simulink model "PSO_ZVD"  (R2021a)
settings: Solver=VariableStepAuto  StartTime=0.0  StopTime=20  RelTol=1e-3
InitFcn:
  | ml=2;
  | 
  | mc=0.5;
  | M2=0.5;
  | 
  | mt=5;
  | g=9.81;
  | l_ref=0.1;
  | l_ini=1;
  | l=l_ini;
  | x_ref=1;
  | n1=5;n2=1;
  | 
  | %ADRC' s parameter caculation
  | %b0 = (ml+mc)/(mc*ml +mc*mt+ml*mt); %Hieu
  | b0=(ml+mc)/(mt*mc+2*ml*mc+mt*ml+ml^2+mc^2); %Enhanced-coupling
  | k_ESO = 100;
  | T_set  = 6;
  | 
  | s_cl = -5.85/T_set;
  | Kp   = s_cl^2;
  | Kd   = -2*s_cl;
  | 
  | s_ESO = k_ESO*s_cl;
  | l1        = -3*s_ESO;
  | l2        = 3*( s_ESO)^2;
  | l3        = -(s_ESO)^3;
  | 
  | %b1 = (mt+mc)/(mc*ml +mc*mt+ml*mt);
  | b1=1/(ml+mc);
  | k_ESO1 =100;
  | T_set1  = 3;
  | s_cl1 = -5.85/T_set1;
  | Kp1   = s_cl1^2;
  | Kd1   = -2*s_cl1;
  | 
  | s_ESO1 = k_ESO1*s_cl1;
  | l11        = -3*s_ESO1;
  | l21        = 3*( s_ESO1)^2;
  | l31        = -(s_ESO1)^3;
  | 
  | 
  | L1=l_ini;
  | %L2=0.5;
  | L2=0.1;
  | m1=2;
  | m2=mc;
  | m=5;
  | %Bo input shaping
  | alpha = (1/L1 + 1/L2)*(m1+M2)/m1;
  | beta = (((m1+M2)/m1)^2)*((1/L1 + 1/L2)^2) - 4*(m1+M2)/(m1*L1*L2);
  | w1 = sqrt(g*(alpha - sqrt(beta))/2);
  | w2 = sqrt(g*(alpha + sqrt(beta))/2);
  | damping_ratio = 0;
  | wd1 = w1*sqrt(1-damping_ratio^2);
  | wd2 = w2*sqrt(1-damping_ratio^2);
  | k = exp(damping_ratio*pi/sqrt(1-damping_ratio^2));
  | 
  | %ZVD1
  | t1_ZVD_1=pi/wd1;
  | ... (+27 lines)
values from neighbouring files (symbols this model uses):
  particle = repmat(empty_particle, nPop, 1)    [PSO16_12.m]    (also in PSO_ZVD.m)
undefined symbols (not defined in the file or in its folder): i, li, xi
libraries: neural x101, simulink_extras x13, simulink x3
(part 23 of 34)

== matlab function PSO_ZVD/non linear model/con lắc đôi4/Crane ==
  data: dx1 output; d1x input; l1 input; d1l1 input; the1 input; d1the1 input; the2 input; d1the2 input; Fx input; Fl input; dx2 output; dx3 output; dx4 output; dx5 output; dx6 output; m2 input; dx7 output; dx8 output
function [dx1,dx2,dx3,dx4,dx5,dx6,dx7,dx8] = fcn(d1x,l1,d1l1,the1,d1the1,the2,d1the2,Fx,Fl,m2)
 m =5; m1 =2; g =9.81; l2=0.5;bx=82; bl=50;bc=0.1;

 dx1=d1x;

 dx2 =(Fx*l1*l2*m2*cos(the1 - the2)^2 - Fx*l1*l2*m2 - d1the2^2*l1*l2^2*m2^2*sin(the2) - Fx*l1*l2*m1 + Fx*l1*l2*m2*sin(the1 - the2)^2 + bx*d1x*l1*l2*m1 + bx*d1x*l1*l2*m2 + Fl*l1*l2*m1*sin(the1) + Fl*l1*l2*m2*sin(the1) - bc*d1the1*l2*m1*cos(the1) - bc*d1the1*l2*m2*cos(the1) - bc*d1the2*l1*m1*cos(the2) - bc*d1the2*l1*m2*cos(the2) + bc*d1the2*l1*m1*sin(the1 - the2)*sin(the1) + bc*d1the2*l1*m2*sin(the1 - the2)*sin(the1) + d1the2^2*l1*l2^2*m2^2*cos(the1 - the2)*sin(the1) - d1the2^2*l1*l2^2*m2^2*sin(the1 - the2)*cos(the1) - d1the2^2*l1*l2^2*m1*m2*sin(the2) - g*l1*l2*m2^2*cos(the2)*sin(the2) - Fl*l1*l2*m2*cos(the1 - the2)^2*sin(the1) + bc*d1the1*l2*m2*sin(the1 - the2)^2*cos(the1) - bl*d1l1*l1*l2*m1*sin(the1) - bl*d1l1*l1*l2*m2*sin(the1) + d1the2^2*l1*l2^2*m2^2*cos(the1 - the2)^2*sin(the2) - d1the2^2*l1*l2^2*m2^2*cos(the1 - the2)^3*sin(the1) + d1the2^2*l1*l2^2*m2^2*sin(the1 - the2)^3*cos(the1) + d1the2^2*l1*l2^2*m2^2*sin(the1 - the2)^2*sin(the2) - bx*d1x*l1*l2*m2*cos(the1 - the2)^2 - Fl*l1*l2*m2*sin(the1 - the2)*cos(the2) + bc*d1the2*l1*m1*cos(the1 - the2)*cos(the1) + bc*d1the2*l1*m2*cos(the1 - the2)*cos(the1) + bc*d1the1*l2*m2*cos(the1 - the2)*cos(the2) - bx*d1x*l1*l2*m2*sin(the1 - the2)^2 - bc*d1the1*l2*m2*cos(the1 - the2)*sin(the1 - the2)*sin(the1) + d1the2^2*l1*l2^2*m1*m2*cos(the1 - the2)*sin(the1) - d1the2^2*l1*l2^2*m1*m2*sin(the1 - the2)*cos(the1) + g*l1*l2*m2^2*cos(the1 - the2)*cos(the1)*sin(the2) + g*l1*l2*m2^2*cos(the1 - the2)*cos(the2)*sin(the1) - g*l1*l2*m2^2*sin(the1 - the2)*cos(the1)*cos(the2) - g*l1*l2*m1*m2*cos(the2)*sin(the2) + g*l1*l2*m2^2*sin(the1 - the2)*sin(the1)*sin(the2) + bl*d1l1*l1*l2*m2*sin(the1 - the2)*cos(the2) + d1the2^2*l1*l2^2*m2^2*cos(the1 - the2)^2*sin(the1 - the2)*cos(the1) - d1the2^2*l1*l2^2*m2^2*cos(the1 - the2)*sin(the1 - the2)^2*sin(the1) - g*l1*l2*m2^2*cos(the1 - the2)^2*cos(the1)*sin(the1) + g*l1*l2*m2^2*sin(the1 - the2)^2*cos(the1)*sin(the1) + bl*d1l1*l1*l2*m2*cos(the1 - the2)^2*sin(the1) + g*l1*l2*m2^2*cos(the1 - the2)*sin(the1 - the2)*cos(the1)^2 - g*l1*l2*m2^2*cos(the1 - the2)*sin(the1 - the2)*sin(the1)^2 + Fl*l1*l2*m2*cos(the1 - the2)*sin(the1 - the2)*cos(the1) + g*l1*l2*m1*m2*cos(the1 - the2)*cos(the1)*sin(the2) + g*l1*l2*m1*m2*cos(the1 - the2)*cos(the2)*sin(the1) - g*l1*l2*m1*m2*sin(the1 - the2)*cos(the1)*cos(the2) + g*l1*l2*m1*m2*sin(the1 - the2)*sin(the1)*sin(the2) - bl*d1l1*l1*l2*m2*cos(the1 - the2)*sin(the1 - the2)*cos(the1) - g*l1*l2*m1*m2*cos(the1 - the2)^2*cos(the1)*sin(the1) + g*l1*l2*m1*m2*sin(the1 - the2)^2*cos(the1)*sin(the1) + g*l1*l2*m1*m2*cos(the1 - the2)*sin(the1 - the2)*cos(the1)^2 - g*l1*l2*m1*m2*cos(the1 - the2)*sin(the1 - the2)*sin(the1)^2)/(l1*l2*(m1^2*cos(the1)^2 - m*m2 - 2*m1*m2 - m*m1 + m2^2*cos(the1)^2 + m2^2*cos(the2)^2 + m1^2*sin(the1)^2 + m2^2*sin(the1)^2 + m2^2*cos(the1 - the2)^2 + m2^2*sin(the1 - the2)^2 - m1^2 - m2^2 + 2*m1*m2*cos(the1)^2 + m1*m2*cos(the2)^2 + 2*m1*m2*sin(the1)^2 + m*m2*cos(the1 - the2)^2 + m1*m2*cos(the1 - the2)^2 + m*m2*sin(the1 - the2)^2 + m1*m2*sin(the1 - the2)^2 - m2^2*cos(the1 - the2)^2*sin(the1)^2 - m2^2*sin(the1 - the2)^2*cos(the1)^2 - 2*m2^2*sin(the1 - the2)*cos(the2)*sin(the1) - 2*m2^2*cos(the1 - the2)*cos(the1)*cos(the2) - m1*m2*cos(the1 - the2)^2*sin(the1)^2 - m1*m2*sin(the1 - the2)^2*cos(the1)^2 + 2*m2^2*cos(the1 - the2)*sin(the1 - the2)*cos(the1)*sin(the1) - 2*m1*m2*sin(the1 - the2)*cos(the2)*sin(the1) - 2*m1*m2*cos(the1 - the2)*cos(the1)*cos(the2) + 2*m1*m2*cos(the1 - the2)*sin(the1 - the2)*cos(the1)*sin(the1)));

 dx3=d1l1;

 dx4 = (Fx*l1*l2*m1^2*sin(the1) - d1the1^2*l1^2*l2*m2^3 - Fl*l1*l2*m1^2 - Fl*l1*l2*m2^2 - d1the2^2*l1*l2^2*m2^3*cos(the1 - the2) - d1the1^2*l1^2*l2*m1^3 + Fx*l1*l2*m2^2*sin(the1) - g*l1*l2*m1^3*cos(the1) - g*l1*l2*m2^3*cos(the1) - Fl*l1*l2*m*m1 - Fl*l1*l2*m*m2 - 2*Fl*l1*l2*m1*m2 + d1the1^2*l1^2*l2*m1^3*cos(the1)^2 + d1the1^2*l1^2*l2*m2^3*cos(the1)^2 + d1the1^2*l1^2*l2*m2^3*cos(the2)^2 + d1the1^2*l1^2*l2*m1^3*sin(the1)^2 + d1the1^2*l1^2*l2*m2^3*sin(the1)^2 - bc*d1the2*l1*m1^2*sin(the1 - the2) - bc*d1the2*l1*m2^2*sin(the1 - the2) + Fl*l1*l2*m1^2*cos(the1)^2 + Fl*l1*l2*m2^2*cos(the1)^2 + Fl*l1*l2*m2^2*cos(the2)^2 + d1the1^2*l1^2*l2*m2^3*cos(the1 - the2)^2 + d1the2^2*l1*l2^2*m2^3*cos(the1 - the2)^3 - d1the1^2*l1^2*l2*m*m1^2 - d1the1^2*l1^2*l2*m*m2^2 - 3*d1the1^2*l1^2*l2*m1*m2^2 - 3*d1the1^2*l1^2*l2*m1^2*m2 + d1the1^2*l1^2*l2*m2^3*sin(the1 - the2)^2 + g*l1*l2*m1^3*cos(the1)^3 + g*l1*l2*m2^3*cos(the1)^3 + Fl*l1*l2*m2^2*cos(the1 - the2)^2 + bl*d1l1*l1*l2*m1^2 + bl*d1l1*l1*l2*m2^2 - bl*d1l1*l1*l2*m1^2*cos(the1)^2 - bl*d1l1*l1*l2*m2^2*cos(the1)^2 - bl*d1l1*l1*l2*m2^2*cos(the2)^2 + d1the1^2*l1^2*l2*m*m2^2*sin(the1 - the2)^2 + 2*d1the1^2*l1^2*l2*m1*m2^2*sin(the1 - the2)^2 + d1the1^2*l1^2*l2*m1^2*m2*sin(the1 - the2)^2 + 3*g*l1*l2*m1*m2^2*cos(the1)^3 + 3*g*l1*l2*m1^2*m2*cos(the1)^3 + bc*d1the1*l2*m1^2*cos(the1)*sin(the1) + bc*d1the1*l2*m2^2*cos(the1)*sin(the1) + bc*d1the2*l1*m1^2*cos(the2)*sin(the1) + bc*d1the2*l1*m2^2*cos(the2)*sin(the1) - bl*d1l1*l1*l2*m2^2*cos(the1 - the2)^2 - Fx*l1*l2*m2^2*sin(the1 - the2)*cos(the2) + 2*Fx*l1*l2*m1*m2*sin(the1) + d1the2^2*l1*l2^2*m2^3*cos(the1 - the2)*cos(the1)^2 + d1the2^2*l1*l2^2*m2^3*cos(the1 - the2)*cos(the2)^2 - g*l1*l2*m2^3*sin(the1 - the2)*sin(the2) + g*l1*l2*m2^3*cos(the1)*cos(the2)^2 + bc*d1the1*l2*m2^2*cos(the1 - the2)*sin(the1 - the2) - bc*d1the2*l1*m*m1*sin(the1 - the2) - bc*d1the2*l1*m*m2*sin(the1 - the2) - 2*bc*d1the2*l1*m1*m2*sin(the1 - the2) + g*l1*l2*m1^3*cos(the1)*sin(the1)^2 + g*l1*l2*m2^3*cos(the1)*sin(the1)^2 + 2*Fl*l1*l2*m1*m2*cos(the1)^2 + Fl*l1*l2*m1*m2*cos(the2)^2 - Fx*l1*l2*m2^2*cos(the1 - the2)^2*sin(the1) - d1the2^2*l1*l2^2*m*m2^2*cos(the1 - the2) - 2*d1the2^2*l1*l2^2*m1*m2^2*cos(the1 - the2) - d1the2^2*l1*l2^2*m1^2*m2*cos(the1 - the2) - 2*d1the1^2*l1^2*l2*m*m1*m2 + d1the2^2*l1*l2^2*m2^3*cos(the1 - the2)*sin(the1 - the2)^2 + g*l1*l2*m2^3*cos(the1 - the2)^2*cos(the1) - g*l1*l2*m*m1^2*cos(the1) - g*l1*l2*m*m2^2*cos(the1) - 3*g*l1*l2*m1*m2^2*cos(the1) - 3*g*l1*l2*m1^2*m2*cos(the1) + bc*d1the2*l1*m1^2*sin(the1 - the2)*cos(the1)^2 + bc*d1the2*l1*m2^2*sin(the1 - the2)*cos(the1)^2 - bx*d1x*l1*l2*m1^2*sin(the1) - bx*d1x*l1*l2*m2^2*sin(the1) + Fl*l1*l2*m*m2*cos(the1 - the2)^2 + Fl*l1*l2*m1*m2*cos(the1 - the2)^2 + 3*d1the1^2*l1^2*l2*m1*m2^2*cos(the1)^2 + 3*d1the1^2*l1^2*l2*m1^2*m2*cos(the1)^2 + 2*d1the1^2*l1^2*l2*m1*m2^2*cos(the2)^2 + d1the1^2*l1^2*l2*m1^2*m2*cos(the2)^2 + bl*d1l1*l1*l2*m*m1 + bl*d1l1*l1*l2*m*m2 + 2*bl*d1l1*l1*l2*m1*m2 - d1the1^2*l1^2*l2*m2^3*cos(the1 - the2)^2*sin(the1)^2 - d1the1^2*l1^2*l2*m2^3*sin(the1 - the2)^2*cos(the1)^2 + 3*d1the1^2*l1^2*l2*m1*m2^2*sin(the1)^2 + 3*d1the1^2*l1^2*l2*m1^2*m2*sin(the1)^2 + d1the2^2*l1*l2^2*m2^3*sin(the1)*sin(the2) + d1the1^2*l1^2*l2*m*m2^2*cos(the1 - the2)^2 + 2*d1the1^2*l1^2*l2*m1*m2^2*cos(the1 - the2)^2 + d1the1^2*l1^2*l2*m1^2*m2*cos(the1 - the2)^2 + d1the2^2*l1*l2^2*m*m2^2*cos(the1 - the2)^3 + d1the2^2*l1*l2^2*m1*m2^2*cos(the1 - the2)^3 - 2*d1the1^2*l1^2*l2*m2^3*sin(the1 - the2)*cos(the2)*sin(the1) + d1the2^2*l1*l2^2*m2^3*sin(the1 - the2)*cos(the1)*sin(the1) - d1the2^2*l1*l2^2*m2^3*sin(the1 - the2)*cos(the2)*sin(the2) - 2*Fl*l1*l2*m2^2*cos(the1 - the2)*cos(the1)*cos(the2) + d1the1^2*l1^2*l2*m*m1*m2*cos(the1 - the2)^2 - 2*bl*d1l1*l1*l2*m1*m2*cos(the1)^2 - bl*d1l1*l1*l2*m1*m2*cos(the2)^2 + g*l1*l2*m2^3*cos(the2)*sin(the1)*sin(the2) + d1the2^2*l1*l2^2*m*m2^2*cos(the1 - the2)*sin(the1 - the2)^2 + d1the2^2*l1*l2^2*m1*m2^2*cos(the1 - the2)*sin(the1 - the2)^2 + g*l1*l2*m*m2^2*cos(the1 - the2)^2*cos(the1) + 2*g*l1*l2*m1*m2^2*cos(the1 - the2)^2*cos(the1) + g*l1*l2*m1^2*m2*cos(the1 - the2)^2*cos(the1) + d1the1^2*l1^2*l2*m*m1*m2*sin(the1 - the2)^2 + bx*d1x*l1*l2*m2^2*cos(the1 - the2)^2*sin(the1) - bc*d1the2*l1*m1^2*cos(the1 - the2)*cos(the1)*sin(the1) - bc*d1the2*l1*m2^2*cos(the1 - the2)*cos(the1)*sin(the1) - bc*d1the1*l2*m2^2*cos(the1 - the2)*cos(the2)*sin(the1) - bc*d1the1*l2*m2^2*sin(the1 - the2)*cos(the1)*cos(the2) + 2*bc*d1the1*l2*m1*m2*cos(the1)*sin(the1) + 2*bc*d1the2*l1*m1*m2*cos(the2)*sin(the1) - 2*d1the2^2*l1*l2^2*m2^3*cos(the1 - the2)^2*cos(the1)*cos(the2) - bl*d1l1*l1*l2*m*m2*cos(the1 - the2)^2 - bl*d1l1*l1*l2*m1*m2*cos(the1 - the2)^2 - 2*d1the1^2*l1^2*l2*m1*m2^2*cos(the1 - the2)^2*sin(the1)^2 - 2*d1the1^2*l1^2*l2*m1*m2^2*sin(the1 - the2)^2*cos(the1)^2 - d1the1^2*l1^2*l2*m1^2*m2*cos(the1 - the2)^2*sin(the1)^2 - d1the1^2*l1^2*l2*m1^2*m2*sin(the1 - the2)^2*cos(the1)^2 + Fx*l1*l2*m2^2*cos(the1 - the2)*sin(the1 - the2)*cos(the1) - Fx*l1*l2*m1*m2*sin(the1 - the2)*cos(the2) - d1the2^2*l1*l2^2*m2^3*sin(the1 - the2)^2*cos(the1)*cos(the2) - d1the2^2*l1*l2^2*m2^3*cos(the1 - the2)^2*sin(the1)*sin(the2) + 2*d1the2^2*l1*l2^2*m1*m2^2*sin(the1)*sin(the2) + d1the2^2*l1*l2^2*m1^2*m2*sin(the1)*sin(the2) + g*l1*l2*m2^3*cos(the1 - the2)*sin(the1 - the2)*sin(the1) - 2*g*l1*l2*m2^3*cos(the1 - the2)*cos(the1)^2*cos(the2) + bc*d1the1*l2*m*m2*cos(the1 - the2)*sin(the1 - the2) + bc*d1the1*l2*m1*m2*cos(the1 - the2)*sin(the1 - the2) - g*l1*l2*m2^3*cos(the1 - the2)*cos(the2)*sin(the1)^2 + g*l1*l2*m2^3*sin(the1 - the2)*cos(the1)^2*sin(the2) - Fx*l1*l2*m1*m2*cos(the1 - the2)^2*sin(the1) - d1the2^2*l1*l2^2*m*m1*m2*cos(the1 - the2) - 2*g*l1*l2*m*m1*m2*cos(the1) + bx*d1x*l1*l2*m2^2*sin(the1 - the2)*cos(the2) + 2*bc*d1the2*l1*m1*m2*sin(the1 - the2)*cos(the1)^2 - 2*bx*d1x*l1*l2*m1*m2*sin(the1) + 2*d1the2^2*l1*l2^2*m1*m2^2*cos(the1 - the2)*cos(the1)^2 + d1the2^2*l1*l2^2*m1^2*m2*cos(the1 - the2)*cos(the1)^2 + d1the2^2*l1*l2^2*m1*m2^2*cos(the1 - the2)*cos(the2)^2 - g*l1*l2*m*m2^2*sin(the1 - the2)*sin(the2) - 2*g*l1*l2*m1*m2^2*sin(the1 - the2)*sin(the2) - g*l1*l2*m1^2*m2*sin(the1 - the2)*sin(the2) - 2*d1the1^2*l1^2*l2*m2^3*cos(the1 - the2)*cos(the1)*cos(the2) + 2*g*l1*l2*m1*m2^2*cos(the1)*cos(the2)^2 + g*l1*l2*m1^2*m2*cos(the1)*cos(the2)^2 + 3*g*l1*l2*m1*m2^2*cos(the1)*sin(the1)^2 + 3*g*l1*l2*m1^2*m2*cos(the1)*sin(the1)^2 - 2*g*l1*l2*m1*m2^2*cos(the1 - the2)*cos(the2)*sin(the1)^2 - g*l1*l2*m1^2*m2*cos(the1 - the2)*cos(the2)*sin(the1)^2 + 2*d1the1^2*l1^2*l2*m2^3*cos(the1 - the2)*sin(the1 - the2)*cos(the1)*sin(the1) + d1the2^2*l1*l2^2*m2^3*cos(the1 - the2)*sin(the1 - the2)*cos(the1)*sin(the2) - d1the2^2*l1*l2^2*m2^3*cos(the1 - the2)*sin(the1 - the2)*cos(the2)*sin(the1) + 2*g*l1*l2*m1*m2^2*sin(the1 - the2)*cos(the1)^2*sin(the2) + g*l1*l2*m1^2*m2*sin(the1 - the2)*cos(the1)^2*sin(the2) - 2*Fl*l1*l2*m1*m2*cos(the1 - the2)*cos(the1)*cos(the2) - g*l1*l2*m2^3*cos(the1 - the2)*cos(the1)*sin(the1)*sin(the2) - g*l1*l2*m2^3*sin(the1 - the2)*cos(the1)*cos(the2)*sin(the1) + g*l1*l2*m*m1*m2*cos(the1 - the2)^2*cos(the1) + bx*d1x*l1*l2*m1*m2*cos(the1 - the2)^2*sin(the1) - 2*bc*d1the2*l1*m1*m2*cos(the1 - the2)*cos(the1)*sin(the1) - bc*d1the1*l2*m1*m2*cos(the1 - the2)*cos(the2)*sin(the1) - bc*d1the1*l2*m1*m2*sin(the1 - the2)*cos(the1)*cos(the2) - 4*d1the1^2*l1^2*l2*m1*m2^2*cos(the1 - the2)*cos(the1)*cos(the2) - 2*d1the1^2*l1^2*l2*m1^2*m2*cos(the1 - the2)*cos(the1)*cos(the2) + Fx*l1*l2*m1*m2*cos(the1 - the2)*sin(the1 - the2)*cos(the1) - 4*d1the1^2*l1^2*l2*m1*m2^2*sin(the1 - the2)*cos(the2)*sin(the1) - 2*d1the1^2*l1^2*l2*m1^2*m2*sin(the1 - the2)*cos(the2)*sin(the1) + 2*d1the2^2*l1*l2^2*m1*m2^2*sin(the1 - the2)*cos(the1)*sin(the1) + d1the2^2*l1*l2^2*m1^2*m2*sin(the1 - the2)*cos(the1)*sin(the1) - d1the2^2*l1*l2^2*m1*m2^2*sin(the1 - the2)*cos(the2)*sin(the2) + 2*g*l1*l2*m1*m2^2*cos(the2)*sin(the1)*sin(the2) + g*l1*l2*m1^2*m2*cos(the2)*sin(the1)*sin(the2) + 2*bl*d1l1*l1*l2*m2^2*cos(the1 - the2)*cos(the1)*cos(the2) - 2*d1the2^2*l1*l2^2*m1*m2^2*cos(the1 - the2)^2*cos(the1)*cos(the2) - d1the2^2*l1*l2^2*m1*m2^2*sin(the1 - the2)^2*cos(the1)*cos(the2) - bx*d1x*l1*l2*m2^2*cos(the1 - the2)*sin(the1 - the2)*cos(the1) + bx*d1x*l1*l2*m1*m2*sin(the1 - the2)*cos(the2) - d1the2^2*l1*l2^2*m1*m2^2*cos(the1 - the2)^2*sin(the1)*sin(the2) + g*l1*l2*m*m2^2*cos(the1 - the2)*sin(the1 - the2)*sin(the1) + 2*g*l1*l2*m1*m2^2*cos(the1 - the2)*sin(the1 - the2)*sin(the1) + g*l1*l2*m1^2*m2*cos(the1 - the2)*sin(the1 - the2)*sin(the1) - g*l1*l2*m*m1*m2*sin(the1 - the2)*sin(the2) - 4*g*l1*l2*m1*m2^2*cos(the1 - the2)*cos(the1)^2*cos(the2) - 2*g*l1*l2*m1^2*m2*cos(the1 - the2)*cos(the1)^2*cos(the2) + 4*d1the1^2*l1^2*l2*m1*m2^2*cos(the1 - the2)*sin(the1 - the2)*cos(the1)*sin(the1) + 2*d1the1^2*l1^2*l2*m1^2*m2*cos(the1 - the2)*sin(the1 - the2)*cos(the1)*sin(the1) + d1the2^2*l1*l2^2*m1*m2^2*cos(the1 - the2)*sin(the1 - the2)*cos(the1)*sin(the2) - d1the2^2*l1*l2^2*m1*m2^2*cos(the1 - the2)*sin(the1 - the2)*cos(the2)*sin(the1) - 2*g*l1*l2*m1*m2^2*cos(the1 - the2)*cos(the1)*sin(the1)*sin(the2) - 2*g*l1*l2*m1*m2^2*sin(the1 - the2)*cos(the1)*cos(the2)*sin(the1) - g*l1*l2*m1^2*m2*cos(the1 - the2)*cos(the1)*sin(the1)*sin(the2) - g*l1*l2*m1^2*m2*sin(the1 - the2)*cos(the1)*cos(the2)*sin(the1) + 2*bl*d1l1*l1*l2*m1*m2*cos(the1 - the2)*cos(the1)*cos(the2) - bx*d1x*l1*l2*m1*m2*cos(the1 - the2)*sin(the1 - the2)*cos(the1) + g*l1*l2*m*m1*m2*cos(the1 - the2)*sin(the1 - the2)*sin(the1))/(l1*l2*(m1 + m2)*(m1^2*cos(the1)^2 - m*m2 - 2*m1*m2 - m*m1 + m2^2*cos(the1)^2 + m2^2*cos(the2)^2 + m1^2*sin(the1)^2 + m2^2*sin(the1)^2 + m2^2*cos(the1 - the2)^2 + m2^2*sin(the1 - the2)^2 - m1^2 - m2^2 + 2*m1*m2*cos(the1)^2 + m1*m2*cos(the2)^2 + 2*m1*m2*sin(the1)^2 + m*m2*cos(the1 - the2)^2 + m1*m2*cos(the1 - the2)^2 + m*m2*sin(the1 - the2)^2 + m1*m2*sin(the1 - the2)^2 - m2^2*cos(the1 - the2)^2*sin(the1)^2 - m2^2*sin(the1 - the2)^2*cos(the1)^2 - 2*m2^2*sin(the1 - the2)*cos(the2)*sin(the1) - 2*m2^2*cos(the1 - the2)*cos(the1)*cos(the2) - m1*m2*cos(the1 - the2)^2*sin(the1)^2 - m1*m2*sin(the1 - the2)^2*cos(the1)^2 + 2*m2^2*cos(the1 - the2)*sin(the1 - the2)*cos(the1)*sin(the1) - 2*m1*m2*sin(the1 - the2)*cos(the2)*sin(the1) - 2*m1*m2*cos(the1 - the2)*cos(the1)*cos(the2) + 2*m1*m2*cos(the1 - the2)*sin(the1 - the2)*cos(the1)*sin(the1)));

 dx5=d1the1;

 dx6 = -(bc*d1the2*l1*m1^2*cos(the1 - the2) - bc*d1the1*l2*m2^2 - Fx*l1*l2*m1^2*cos(the1) - Fx*l1*l2*m2^2*cos(the1) - d1the2^2*l1*l2^2*m2^3*sin(the1 - the2) - g*l1*l2*m1^3*sin(the1) - g*l1*l2*m2^3*sin(the1) - bc*d1the1*l2*m1^2 + bc*d1the2*l1*m2^2*cos(the1 - the2) - bc*d1the1*l2*m*m1 - bc*d1the1*l2*m*m2 - 2*bc*d1the1*l2*m1*m2 + bc*d1the1*l2*m2^2*cos(the2)^2 + d1the2^2*l1*l2^2*m2^3*sin(the1 - the2)^3 + bc*d1the1*l2*m1^2*sin(the1)^2 + bc*d1the1*l2*m2^2*sin(the1)^2 + g*l1*l2*m1^3*sin(the1)^3 + g*l1*l2*m2^3*sin(the1)^3 - 2*d1l1*d1the1*l1*l2*m1^3 - 2*d1l1*d1the1*l1*l2*m2^3 + bc*d1the1*l2*m2^2*sin(the1 - the2)^2 + 2*d1l1*d1the1*l1*l2*m1^3*cos(the1)^2 + 2*d1l1*d1the1*l1*l2*m2^3*cos(the1)^2 + 2*d1l1*d1the1*l1*l2*m2^3*cos(the2)^2 + Fl*l1*l2*m1^2*cos(the1)*sin(the1) + Fl*l1*l2*m2^2*cos(the1)*sin(the1) - bc*d1the2*l1*m1^2*cos(the1)*cos(the2) - bc*d1the2*l1*m2^2*cos(the1)*cos(the2) + d1the2^2*l1*l2^2*m*m2^2*sin(the1 - the2)^3 + d1the2^2*l1*l2^2*m1*m2^2*sin(the1 - the2)^3 + 2*d1l1*d1the1*l1*l2*m1^3*sin(the1)^2 + 2*d1l1*d1the1*l1*l2*m2^3*sin(the1)^2 + 3*g*l1*l2*m1*m2^2*sin(the1)^3 + 3*g*l1*l2*m1^2*m2*sin(the1)^3 + Fx*l1*l2*m2^2*cos(the1 - the2)*cos(the2) - 2*Fx*l1*l2*m1*m2*cos(the1) + 2*d1l1*d1the1*l1*l2*m2^3*cos(the1 - the2)^2 - 2*d1l1*d1the1*l1*l2*m*m1^2 - 2*d1l1*d1the1*l1*l2*m*m2^2 - 6*d1l1*d1the1*l1*l2*m1*m2^2 - 6*d1l1*d1the1*l1*l2*m1^2*m2 + 2*d1l1*d1the1*l1*l2*m2^3*sin(the1 - the2)^2 + g*l1*l2*m2^3*cos(the1 - the2)*sin(the2) + Fl*l1*l2*m2^2*cos(the1 - the2)*sin(the1 - the2) + bc*d1the2*l1*m*m1*cos(the1 - the2) + bc*d1the2*l1*m*m2*cos(the1 - the2) + 2*bc*d1the2*l1*m1*m2*cos(the1 - the2) + d1the2^2*l1*l2^2*m2^3*sin(the1 - the2)*cos(the2)^2 + d1the2^2*l1*l2^2*m2^3*sin(the1 - the2)*sin(the1)^2 + g*l1*l2*m1^3*cos(the1)^2*sin(the1) + g*l1*l2*m2^3*cos(the1)^2*sin(the1) + g*l1*l2*m2^3*cos(the2)^2*sin(the1) + Fx*l1*l2*m2^2*sin(the1 - the2)^2*cos(the1) + bx*d1x*l1*l2*m1^2*cos(the1) + bx*d1x*l1*l2*m2^2*cos(the1) + bc*d1the1*l2*m1*m2*cos(the2)^2 + d1the2^2*l1*l2^2*m2^3*cos(the1 - the2)^2*sin(the1 - the2) - d1the2^2*l1*l2^2*m*m2^2*sin(the1 - the2) - 2*d1the2^2*l1*l2^2*m1*m2^2*sin(the1 - the2) - d1the2^2*l1*l2^2*m1^2*m2*sin(the1 - the2) - bc*d1the2*l1*m1^2*cos(the1 - the2)*sin(the1)^2 - bc*d1the2*l1*m2^2*cos(the1 - the2)*sin(the1)^2 + 2*bc*d1the1*l2*m1*m2*sin(the1)^2 - g*l1*l2*m*m1^2*sin(the1) - g*l1*l2*m*m2^2*sin(the1) - 3*g*l1*l2*m1*m2^2*sin(the1) - 3*g*l1*l2*m1^2*m2*sin(the1) + g*l1*l2*m2^3*sin(the1 - the2)^2*sin(the1) + bc*d1the1*l2*m*m2*sin(the1 - the2)^2 + bc*d1the1*l2*m1*m2*sin(the1 - the2)^2 - d1the2^2*l1*l2^2*m2^3*cos(the1)*sin(the2) - g*l1*l2*m2^3*cos(the1)*cos(the2)*sin(the2) - Fl*l1*l2*m2^2*cos(the1 - the2)*cos(the2)*sin(the1) - Fl*l1*l2*m2^2*sin(the1 - the2)*cos(the1)*cos(the2) + 2*Fl*l1*l2*m1*m2*cos(the1)*sin(the1) + d1the2^2*l1*l2^2*m*m2^2*cos(the1 - the2)^2*sin(the1 - the2) + d1the2^2*l1*l2^2*m1*m2^2*cos(the1 - the2)^2*sin(the1 - the2) - 2*bc*d1the2*l1*m1*m2*cos(the1)*cos(the2) - bx*d1x*l1*l2*m2^2*sin(the1 - the2)^2*cos(the1) + bc*d1the2*l1*m1^2*sin(the1 - the2)*cos(the1)*sin(the1) + bc*d1the2*l1*m2^2*sin(the1 - the2)*cos(the1)*sin(the1) - 2*bc*d1the1*l2*m2^2*sin(the1 - the2)*cos(the2)*sin(the1) + g*l1*l2*m*m2^2*sin(the1 - the2)^2*sin(the1) + 2*g*l1*l2*m1*m2^2*sin(the1 - the2)^2*sin(the1) + g*l1*l2*m1^2*m2*sin(the1 - the2)^2*sin(the1) + Fx*l1*l2*m1*m2*cos(the1 - the2)*cos(the2) - 4*d1l1*d1the1*l1*l2*m*m1*m2 - d1the2^2*l1*l2^2*m2^3*cos(the1 - the2)^2*cos(the2)*sin(the1) - 2*d1the2^2*l1*l2^2*m1*m2^2*cos(the1)*sin(the2) - d1the2^2*l1*l2^2*m1^2*m2*cos(the1)*sin(the2) - Fx*l1*l2*m2^2*cos(the1 - the2)*sin(the1 - the2)*sin(the1) + d1the2^2*l1*l2^2*m2^3*sin(the1 - the2)^2*cos(the1)*sin(the2) - 2*d1the2^2*l1*l2^2*m2^3*sin(the1 - the2)^2*cos(the2)*sin(the1) + g*l1*l2*m2^3*cos(the1 - the2)*sin(the1 - the2)*cos(the1) + 6*d1l1*d1the1*l1*l2*m1*m2^2*cos(the1)^2 + 6*d1l1*d1the1*l1*l2*m1^2*m2*cos(the1)^2 + 4*d1l1*d1the1*l1*l2*m1*m2^2*cos(the2)^2 + 2*d1l1*d1the1*l1*l2*m1^2*m2*cos(the2)^2 - 2*d1l1*d1the1*l1*l2*m2^3*cos(the1 - the2)^2*sin(the1)^2 - 2*d1l1*d1the1*l1*l2*m2^3*sin(the1 - the2)^2*cos(the1)^2 + Fl*l1*l2*m*m2*cos(the1 - the2)*sin(the1 - the2) + Fl*l1*l2*m1*m2*cos(the1 - the2)*sin(the1 - the2) + 6*d1l1*d1the1*l1*l2*m1*m2^2*sin(the1)^2 + 6*d1l1*d1the1*l1*l2*m1^2*m2*sin(the1)^2 - bl*d1l1*l1*l2*m1^2*cos(the1)*sin(the1) - bl*d1l1*l1*l2*m2^2*cos(the1)*sin(the1) - g*l1*l2*m2^3*sin(the1 - the2)*cos(the1)^2*cos(the2) + 2*d1l1*d1the1*l1*l2*m*m2^2*cos(the1 - the2)^2 + 4*d1l1*d1the1*l1*l2*m1*m2^2*cos(the1 - the2)^2 + 2*d1l1*d1the1*l1*l2*m1^2*m2*cos(the1 - the2)^2 - g*l1*l2*m2^3*cos(the1 - the2)*sin(the1)^2*sin(the2) - 2*g*l1*l2*m2^3*sin(the1 - the2)*cos(the2)*sin(the1)^2 + Fx*l1*l2*m1*m2*sin(the1 - the2)^2*cos(the1) - bx*d1x*l1*l2*m2^2*cos(the1 - the2)*cos(the2) + 2*bx*d1x*l1*l2*m1*m2*cos(the1) + 2*d1l1*d1the1*l1*l2*m*m2^2*sin(the1 - the2)^2 + 4*d1l1*d1the1*l1*l2*m1*m2^2*sin(the1 - the2)^2 + 2*d1l1*d1the1*l1*l2*m1^2*m2*sin(the1 - the2)^2 - d1the2^2*l1*l2^2*m*m1*m2*sin(the1 - the2) - 2*bc*d1the2*l1*m1*m2*cos(the1 - the2)*sin(the1)^2 + g*l1*l2*m*m2^2*cos(the1 - the2)*sin(the2) + 2*g*l1*l2*m1*m2^2*cos(the1 - the2)*sin(the2) + g*l1*l2*m1^2*m2*cos(the1 - the2)*sin(the2) - 2*g*l1*l2*m*m1*m2*sin(the1) + d1the2^2*l1*l2^2*m1*m2^2*sin(the1 - the2)*cos(the2)^2 - bl*d1l1*l1*l2*m2^2*cos(the1 - the2)*sin(the1 - the2) + d1the2^2*l1*l2^2*m2^3*cos(the1 - the2)*cos(the1)*sin(the1) + d1the2^2*l1*l2^2*m2^3*cos(the1 - the2)*cos(the2)*sin(the2) + 2*d1the2^2*l1*l2^2*m1*m2^2*sin(the1 - the2)*sin(the1)^2 + d1the2^2*l1*l2^2*m1^2*m2*sin(the1 - the2)*sin(the1)^2 + 3*g*l1*l2*m1*m2^2*cos(the1)^2*sin(the1) + 3*g*l1*l2*m1^2*m2*cos(the1)^2*sin(the1) + 2*g*l1*l2*m1*m2^2*cos(the2)^2*sin(the1) + g*l1*l2*m1^2*m2*cos(the2)^2*sin(the1) - 2*g*l1*l2*m1*m2^2*sin(the1 - the2)*cos(the1)^2*cos(the2) - g*l1*l2*m1^2*m2*sin(the1 - the2)*cos(the1)^2*cos(the2) - g*l1*l2*m2^3*cos(the1 - the2)*cos(the1)*cos(the2)*sin(the1) - 2*g*l1*l2*m1*m2^2*cos(the1 - the2)*sin(the1)^2*sin(the2) - 4*g*l1*l2*m1*m2^2*sin(the1 - the2)*cos(the2)*sin(the1)^2 - g*l1*l2*m1^2*m2*cos(the1 - the2)*sin(the1)^2*sin(the2) - 2*g*l1*l2*m1^2*m2*sin(the1 - the2)*cos(the2)*sin(the1)^2 - d1the2^2*l1*l2^2*m2^3*cos(the1 - the2)*sin(the1 - the2)*sin(the1)*sin(the2) - Fl*l1*l2*m1*m2*cos(the1 - the2)*cos(the2)*sin(the1) - Fl*l1*l2*m1*m2*sin(the1 - the2)*cos(the1)*cos(the2) - bx*d1x*l1*l2*m1*m2*sin(the1 - the2)^2*cos(the1) + g*l1*l2*m2^3*sin(the1 - the2)*cos(the1)*sin(the1)*sin(the2) + 2*bc*d1the2*l1*m1*m2*sin(the1 - the2)*cos(the1)*sin(the1) - 2*bc*d1the1*l2*m1*m2*sin(the1 - the2)*cos(the2)*sin(the1) + g*l1*l2*m*m1*m2*sin(the1 - the2)^2*sin(the1) + 2*d1the2^2*l1*l2^2*m1*m2^2*cos(the1 - the2)*cos(the1)*sin(the1) + d1the2^2*l1*l2^2*m1^2*m2*cos(the1 - the2)*cos(the1)*sin(the1) + d1the2^2*l1*l2^2*m1*m2^2*cos(the1 - the2)*cos(the2)*sin(the2) - Fx*l1*l2*m1*m2*cos(the1 - the2)*sin(the1 - the2)*sin(the1) - 2*g*l1*l2*m1*m2^2*cos(the1)*cos(the2)*sin(the2) - g*l1*l2*m1^2*m2*cos(the1)*cos(the2)*sin(the2) - 4*d1l1*d1the1*l1*l2*m2^3*cos(the1 - the2)*cos(the1)*cos(the2) + bl*d1l1*l1*l2*m2^2*cos(the1 - the2)*cos(the2)*sin(the1) + bl*d1l1*l1*l2*m2^2*sin(the1 - the2)*cos(the1)*cos(the2) - 2*bl*d1l1*l1*l2*m1*m2*cos(the1)*sin(the1) - 4*d1l1*d1the1*l1*l2*m2^3*sin(the1 - the2)*cos(the2)*sin(the1) + 2*d1l1*d1the1*l1*l2*m*m1*m2*cos(the1 - the2)^2 - bx*d1x*l1*l2*m1*m2*cos(the1 - the2)*cos(the2) - d1the2^2*l1*l2^2*m1*m2^2*cos(the1 - the2)^2*cos(the2)*sin(the1) + 2*d1l1*d1the1*l1*l2*m*m1*m2*sin(the1 - the2)^2 + d1the2^2*l1*l2^2*m1*m2^2*sin(the1 - the2)^2*cos(the1)*sin(the2) - 2*d1the2^2*l1*l2^2*m1*m2^2*sin(the1 - the2)^2*cos(the2)*sin(the1) + g*l1*l2*m*m2^2*cos(the1 - the2)*sin(the1 - the2)*cos(the1) + 2*g*l1*l2*m1*m2^2*cos(the1 - the2)*sin(the1 - the2)*cos(the1) + g*l1*l2*m1^2*m2*cos(the1 - the2)*sin(the1 - the2)*cos(the1) + g*l1*l2*m*m1*m2*cos(the1 - the2)*sin(the2) + bx*d1x*l1*l2*m2^2*cos(the1 - the2)*sin(the1 - the2)*sin(the1) - 4*d1l1*d1the1*l1*l2*m1*m2^2*cos(the1 - the2)^2*sin(the1)^2 - 4*d1l1*d1the1*l1*l2*m1*m2^2*sin(the1 - the2)^2*cos(the1)^2 - 2*d1l1*d1the1*l1*l2*m1^2*m2*cos(the1 - the2)^2*sin(the1)^2 - 2*d1l1*d1the1*l1*l2*m1^2*m2*sin(the1 - the2)^2*cos(the1)^2 - d1the2^2*l1*l2^2*m2^3*cos(the1 - the2)*sin(the1 - the2)*cos(the1)*cos(the2) - bl*d1l1*l1*l2*m*m2*cos(the1 - the2)*sin(the1 - the2) - bl*d1l1*l1*l2*m1*m2*cos(the1 - the2)*sin(the1 - the2) - 8*d1l1*d1the1*l1*l2*m1*m2^2*sin(the1 - the2)*cos(the2)*sin(the1) - 4*d1l1*d1the1*l1*l2*m1^2*m2*sin(the1 - the2)*cos(the2)*sin(the1) - d1the2^2*l1*l2^2*m1*m2^2*cos(the1 - the2)*sin(the1 - the2)*cos(the1)*cos(the2) - 2*g*l1*l2*m1*m2^2*cos(the1 - the2)*cos(the1)*cos(the2)*sin(the1) - g*l1*l2*m1^2*m2*cos(the1 - the2)*cos(the1)*cos(the2)*sin(the1) - d1the2^2*l1*l2^2*m1*m2^2*cos(the1 - the2)*sin(the1 - the2)*sin(the1)*sin(the2) + 2*g*l1*l2*m1*m2^2*sin(the1 - the2)*cos(the1)*sin(the1)*sin(the2) + g*l1*l2*m1^2*m2*sin(the1 - the2)*cos(the1)*sin(the1)*sin(the2) + bl*d1l1*l1*l2*m1*m2*cos(the1 - the2)*cos(the2)*sin(the1) + bl*d1l1*l1*l2*m1*m2*sin(the1 - the2)*cos(the1)*cos(the2) + 4*d1l1*d1the1*l1*l2*m2^3*cos(the1 - the2)*sin(the1 - the2)*cos(the1)*sin(the1) + g*l1*l2*m*m1*m2*cos(the1 - the2)*sin(the1 - the2)*cos(the1) + bx*d1x*l1*l2*m1*m2*cos(the1 - the2)*sin(the1 - the2)*sin(the1) - 8*d1l1*d1the1*l1*l2*m1*m2^2*cos(the1 - the2)*cos(the1)*cos(the2) - 4*d1l1*d1the1*l1*l2*m1^2*m2*cos(the1 - the2)*cos(the1)*cos(the2) + 8*d1l1*d1the1*l1*l2*m1*m2^2*cos(the1 - the2)*sin(the1 - the2)*cos(the1)*sin(the1) + 4*d1l1*d1the1*l1*l2*m1^2*m2*cos(the1 - the2)*sin(the1 - the2)*cos(the1)*sin(the1))/(l1^2*l2*(m1 + m2)*(m1^2*cos(the1)^2 - m*m2 - 2*m1*m2 - m*m1 + m2^2*cos(the1)^2 + m2^2*cos(the2)^2 + m1^2*sin(the1)^2 + m2^2*sin(the1)^2 + m2^2*cos(the1 - the2)^2 + m2^2*sin(the1 - the2)^2 - m1^2 - m2^2 + 2*m1*m2*cos(the1)^2 + m1*m2*cos(the2)^2 + 2*m1*m2*sin(the1)^2 + m*m2*cos(the1 - the2)^2 + m1*m2*cos(the1 - the2)^2 + m*m2*sin(the1 - the2)^2 + m1*m2*sin(the1 - the2)^2 - m2^2*cos(the1 - the2)^2*sin(the1)^2 - m2^2*sin(the1 - the2)^2*cos(the1)^2 - 2*m2^2*sin(the1 - the2)*cos(the2)*sin(the1) - 2*m2^2*cos(the1 - the2)*cos(the1)*cos(the2) - m1*m2*cos(the1 - the2)^2*sin(the1)^2 - m1*m2*sin(the1 - the2)^2*cos(the1)^2 + 2*m2^2*cos(the1 - the2)*sin(the1 - the2)*cos(the1)*sin(the1) - 2*m1*m2*sin(the1 - the2)*cos(the2)*sin(the1) - 2*m1*m2*cos(the1 - the2)*cos(the1)*cos(the2) + 2*m1*m2*cos(the1 - the2)*sin(the1 - the2)*cos(the1)*sin(the1)));
 
 dx7=d1the2;

 dx8 = -(bc*d1the1*l2*m2^2*cos(the1 - the2) - bc*d1the2*l1*m2^2 - Fx*l1*l2*m2^2*cos(the2) - g*l1*l2*m2^3*sin(the2) - Fl*l1*l2*m2^2*sin(the1 - the2) - bc*d1the2*l1*m1^2 - bc*d1the2*l1*m*m1 - bc*d1the2*l1*m*m2 - 2*bc*d1the2*l1*m1*m2 + bc*d1the2*l1*m1^2*cos(the1)^2 + bc*d1the2*l1*m2^2*cos(the1)^2 + bc*d1the2*l1*m1^2*sin(the1)^2 + bc*d1the2*l1*m2^2*sin(the1)^2 + Fl*l1*l2*m2^2*cos(the2)*sin(the1) - bc*d1the1*l2*m2^2*cos(the1)*cos(the2) + Fx*l1*l2*m2^2*cos(the1 - the2)*cos(the1) - Fx*l1*l2*m1*m2*cos(the2) + Fx*l1*l2*m2^2*sin(the1 - the2)*sin(the1) + g*l1*l2*m2^3*cos(the1 - the2)*sin(the1) - g*l1*l2*m2^3*sin(the1 - the2)*cos(the1) - Fl*l1*l2*m*m2*sin(the1 - the2) - Fl*l1*l2*m1*m2*sin(the1 - the2) + bc*d1the1*l2*m*m2*cos(the1 - the2) + bc*d1the1*l2*m1*m2*cos(the1 - the2) + g*l1*l2*m2^3*cos(the1)^2*sin(the2) + g*l1*l2*m2^3*sin(the1)^2*sin(the2) + Fl*l1*l2*m2^2*sin(the1 - the2)*cos(the1)^2 + bx*d1x*l1*l2*m2^2*cos(the2) + 2*bc*d1the2*l1*m1*m2*cos(the1)^2 - bc*d1the1*l2*m2^2*cos(the1 - the2)*sin(the1)^2 + 2*bc*d1the2*l1*m1*m2*sin(the1)^2 - g*l1*l2*m2^3*cos(the1 - the2)*sin(the1)^3 + g*l1*l2*m2^3*sin(the1 - the2)*cos(the1)^3 - g*l1*l2*m*m2^2*sin(the2) - 2*g*l1*l2*m1*m2^2*sin(the2) - g*l1*l2*m1^2*m2*sin(the2) + bl*d1l1*l1*l2*m2^2*sin(the1 - the2) - d1the2^2*l1*l2^2*m2^3*cos(the2)*sin(the2) + 2*g*l1*l2*m1*m2^2*sin(the1)^2*sin(the2) + g*l1*l2*m1^2*m2*sin(the1)^2*sin(the2) + d1the2^2*l1*l2^2*m2^3*sin(the1 - the2)*sin(the1)*sin(the2) - Fl*l1*l2*m2^2*cos(the1 - the2)*cos(the1)*sin(the1) + Fl*l1*l2*m1*m2*cos(the2)*sin(the1) - bc*d1the1*l2*m1*m2*cos(the1)*cos(the2) - bl*d1l1*l1*l2*m2^2*sin(the1 - the2)*cos(the1)^2 - 2*g*l1*l2*m1*m2^2*cos(the1 - the2)*sin(the1)^3 + 2*g*l1*l2*m1*m2^2*sin(the1 - the2)*cos(the1)^3 - g*l1*l2*m1^2*m2*cos(the1 - the2)*sin(the1)^3 + g*l1*l2*m1^2*m2*sin(the1 - the2)*cos(the1)^3 + bc*d1the1*l2*m2^2*sin(the1 - the2)*cos(the1)*sin(the1) + Fx*l1*l2*m1*m2*cos(the1 - the2)*cos(the1) - d1the2^2*l1*l2^2*m2^3*cos(the1 - the2)^2*cos(the1)*sin(the1) - d1the2^2*l1*l2^2*m1*m2^2*cos(the2)*sin(the2) + Fx*l1*l2*m1*m2*sin(the1 - the2)*sin(the1) + d1the2^2*l1*l2^2*m2^3*sin(the1 - the2)^2*cos(the1)*sin(the1) + d1the2^2*l1*l2^2*m2^3*cos(the1 - the2)*sin(the1 - the2)*cos(the1)^2 - bl*d1l1*l1*l2*m2^2*cos(the2)*sin(the1) - d1the2^2*l1*l2^2*m2^3*cos(the1 - the2)*sin(the1 - the2)*sin(the1)^2 - g*l1*l2*m2^3*cos(the1 - the2)*cos(the1)^2*sin(the1) + g*l1*l2*m2^3*sin(the1 - the2)*cos(the1)*sin(the1)^2 + Fl*l1*l2*m1*m2*sin(the1 - the2)*cos(the1)^2 - bx*d1x*l1*l2*m2^2*cos(the1 - the2)*cos(the1) + bx*d1x*l1*l2*m1*m2*cos(the2) - bc*d1the1*l2*m1*m2*cos(the1 - the2)*sin(the1)^2 + g*l1*l2*m*m2^2*cos(the1 - the2)*sin(the1) - g*l1*l2*m*m2^2*sin(the1 - the2)*cos(the1) + 2*g*l1*l2*m1*m2^2*cos(the1 - the2)*sin(the1) - 2*g*l1*l2*m1*m2^2*sin(the1 - the2)*cos(the1) + g*l1*l2*m1^2*m2*cos(the1 - the2)*sin(the1) - g*l1*l2*m1^2*m2*sin(the1 - the2)*cos(the1) - g*l1*l2*m*m1*m2*sin(the2) - bx*d1x*l1*l2*m2^2*sin(the1 - the2)*sin(the1) + d1the2^2*l1*l2^2*m2^3*cos(the1 - the2)*cos(the1)*sin(the2) + d1the2^2*l1*l2^2*m2^3*cos(the1 - the2)*cos(the2)*sin(the1) - d1the2^2*l1*l2^2*m2^3*sin(the1 - the2)*cos(the1)*cos(the2) + bl*d1l1*l1*l2*m*m2*sin(the1 - the2) + bl*d1l1*l1*l2*m1*m2*sin(the1 - the2) + 2*g*l1*l2*m1*m2^2*cos(the1)^2*sin(the2) + g*l1*l2*m1^2*m2*cos(the1)^2*sin(the2) - d1the2^2*l1*l2^2*m1*m2^2*cos(the1 - the2)*sin(the1 - the2)*sin(the1)^2 - 2*g*l1*l2*m1*m2^2*cos(the1 - the2)*cos(the1)^2*sin(the1) - g*l1*l2*m1^2*m2*cos(the1 - the2)*cos(the1)^2*sin(the1) + 2*g*l1*l2*m1*m2^2*sin(the1 - the2)*cos(the1)*sin(the1)^2 + g*l1*l2*m1^2*m2*sin(the1 - the2)*cos(the1)*sin(the1)^2 - Fl*l1*l2*m1*m2*cos(the1 - the2)*cos(the1)*sin(the1) - bl*d1l1*l1*l2*m1*m2*sin(the1 - the2)*cos(the1)^2 + bc*d1the1*l2*m1*m2*sin(the1 - the2)*cos(the1)*sin(the1) + d1the2^2*l1*l2^2*m1*m2^2*cos(the1 - the2)*cos(the1)*sin(the2) + d1the2^2*l1*l2^2*m1*m2^2*cos(the1 - the2)*cos(the2)*sin(the1) - d1the2^2*l1*l2^2*m1*m2^2*sin(the1 - the2)*cos(the1)*cos(the2) + d1the2^2*l1*l2^2*m1*m2^2*sin(the1 - the2)*sin(the1)*sin(the2) + bl*d1l1*l1*l2*m2^2*cos(the1 - the2)*cos(the1)*sin(the1) - bl*d1l1*l1*l2*m1*m2*cos(the2)*sin(the1) - bx*d1x*l1*l2*m1*m2*cos(the1 - the2)*cos(the1) - d1the2^2*l1*l2^2*m1*m2^2*cos(the1 - the2)^2*cos(the1)*sin(the1) + d1the2^2*l1*l2^2*m1*m2^2*sin(the1 - the2)^2*cos(the1)*sin(the1) + g*l1*l2*m*m1*m2*cos(the1 - the2)*sin(the1) - g*l1*l2*m*m1*m2*sin(the1 - the2)*cos(the1) - bx*d1x*l1*l2*m1*m2*sin(the1 - the2)*sin(the1) + d1the2^2*l1*l2^2*m1*m2^2*cos(the1 - the2)*sin(the1 - the2)*cos(the1)^2 + bl*d1l1*l1*l2*m1*m2*cos(the1 - the2)*cos(the1)*sin(the1))/(l1*l2^2*m2*(m1^2*cos(the1)^2 - m*m2 - 2*m1*m2 - m*m1 + m2^2*cos(the1)^2 + m2^2*cos(the2)^2 + m1^2*sin(the1)^2 + m2^2*sin(the1)^2 + m2^2*cos(the1 - the2)^2 + m2^2*sin(the1 - the2)^2 - m1^2 - m2^2 + 2*m1*m2*cos(the1)^2 + m1*m2*cos(the2)^2 + 2*m1*m2*sin(the1)^2 + m*m2*cos(the1 - the2)^2 + m1*m2*cos(the1 - the2)^2 + m*m2*sin(the1 - the2)^2 + m1*m2*sin(the1 - the2)^2 - m2^2*cos(the1 - the2)^2*sin(the1)^2 - m2^2*sin(the1 - the2)^2*cos(the1)^2 - 2*m2^2*sin(the1 - the2)*cos(the2)*sin(the1) - 2*m2^2*cos(the1 - the2)*cos(the1)*cos(the2) - m1*m2*cos(the1 - the2)^2*sin(the1)^2 - m1*m2*sin(the1 - the2)^2*cos(the1)^2 + 2*m2^2*cos(the1 - the2)*sin(the1 - the2)*cos(the1)*sin(the1) - 2*m1*m2*sin(the1 - the2)*cos(the2)*sin(the1) - 2*m1*m2*cos(the1 - the2)*cos(the1)*cos(the2) + 2*m1*m2*cos(the1 - the2)*sin(the1 - the2)*cos(the1)*sin(the1)));

== matlab function PSO_ZVD/non linear model/Model_Baocao/Crane ==
  data: d1x input; l input; d1l input; the input; dx1 output; d1the input; Fx input; Fl input; dx2 output; dx3 output; dx4 output; dx5 output; dx6 output; bc input; mp input
function [dx1,dx2,dx3,dx4,dx5,dx6] = fcn(d1x,l,d1l,the,d1the,Fx,Fl,bc,mp)
 mt =5; mh =2; bt =0; br =0;  g =9.81;
 %bt =20; br =50;

dx1 = d1x;
dx2 = (Fx*l*mh + Fx*l*mp - Fl*l*mp*sin(the) + bc*d1the*mh*cos(the) + bc*d1the*mp*cos(the) - d1the^2*l^2*mp^2*sin(the) + d1x^2*l^2*mp^2*sin(the) - bt*d1x*l*mh - bt*d1x*l*mp + d1x^2*l^2*mh*mp*sin(the) + br*d1l*l*mp*sin(the) + g*l*mh*mp*cos(the)*sin(the))/(l*(mh*mp + mh*mt + mp*mt - mp^2*cos(the)^2 - mp^2*sin(the)^2 + mp^2 - mh*mp*cos(the)^2));
%dx2= -(bt*x2*mc - ml*ut - mc*ul*sin(x5) - mc*ut + bt*x2*ml - x6^2*x3*mc^2*sin(x5) + br*x4*mc*sin(x5) + Dt*x6*mc^2*cos(x5) + x6^2*x3*mc*ml*sin(x5) + g*mc*ml*cos(x5)*sin(x5) + Dt*x6*mc*ml*cos(x5))/(mc*ml + mc*mt + ml*mt - mc^2*cos(x5)^2 - mc^2*sin(x5)^2 + mc^2 - mc*ml*cos(x5)^2);
 
dx3 = d1l;
dx4 = -(d1x^2*l^2*mp^2*sin(the)^2 - Fl*l*mt - d1the^2*l^2*mp^2 - Fl*l*mp + g*l*mp^2*cos(the)^3 + Fx*l*mp*sin(the) + Fl*l*mp*cos(the)^2 - d1the^2*l^2*mp*mt - g*l*mp^2*cos(the) + d1the^2*l^2*mp^2*cos(the)^2 + br*d1l*l*mp + br*d1l*l*mt + g*l*mp^2*cos(the)*sin(the)^2 - br*d1l*l*mp*cos(the)^2 + bc*d1the*mp*cos(the)*sin(the) - g*l*mp*mt*cos(the) - bt*d1x*l*mp*sin(the))/(l*(mh*mp + mh*mt + mp*mt - mp^2*cos(the)^2 - mp^2*sin(the)^2 + mp^2 - mh*mp*cos(the)^2));
%dx4 = -(mc*ul*cos(x5)^2 - mt*ul - mc*ut*sin(x5) - 2*x6^2*x3*mc^2 - g*mc^2*cos(x5) - mc*ul + br*x4*mc + br*x4*mt + g*mc^2*cos(x5)^3 - 2*x6^2*x3*mc*mt - g*mc*mt*cos(x5) + bt*x2*mc*sin(x5) + 2*x6^2*x3*mc^2*cos(x5)^2 + x6^2*x3*mc^2*sin(x5)^2 + g*mc^2*cos(x5)*sin(x5)^2 - br*x4*mc*cos(x5)^2 + Dt*x6*mc^2*cos(x5)*sin(x5))/(mc*ml + mc*mt + ml*mt - mc^2*cos(x5)^2 - mc^2*sin(x5)^2 + mc^2 - mc*ml*cos(x5)^2);
dx5 = d1the;
dx6 = -(bc*d1the*mp^2 + bc*d1the*mh*mp + bc*d1the*mh*mt + bc*d1the*mp*mt - bc*d1the*mp^2*sin(the)^2 - g*l*mp^3*sin(the)^3 + 2*d1l*d1the*l*mp^3 + Fx*l*mp^2*cos(the) + g*l*mp^3*sin(the) - g*l*mp^3*cos(the)^2*sin(the) - bt*d1x*l*mp^2*cos(the) + g*l*mh*mp^2*sin(the) + g*l*mp^2*mt*sin(the) - d1the^2*l^2*mp^3*cos(the)*sin(the) + d1x^2*l^2*mp^3*cos(the)*sin(the) - 2*d1l*d1the*l*mp^3*cos(the)^2 - Fl*l*mp^2*cos(the)*sin(the) - 2*d1l*d1the*l*mp^3*sin(the)^2 + Fx*l*mh*mp*cos(the) + 2*d1l*d1the*l*mh*mp^2 + 2*d1l*d1the*l*mp^2*mt - 2*d1l*d1the*l*mh*mp^2*cos(the)^2 + br*d1l*l*mp^2*cos(the)*sin(the) - bt*d1x*l*mh*mp*cos(the) + g*l*mh*mp*mt*sin(the) + 2*d1l*d1the*l*mh*mp*mt + d1x^2*l^2*mh*mp^2*cos(the)*sin(the))/(l^2*mp*(mh*mp + mh*mt + mp*mt - mp^2*cos(the)^2 - mp^2*sin(the)^2 + mp^2 - mh*mp*cos(the)^2));
%dx6 = -(g*mc^2*sin(x5) - ml*ut*cos(x5) - mc*ut*cos(x5) + Dt*x6*mc^2 - g*mc^2*sin(x5)^3 + 2*x4*x6*mc^2 - mc*ul*cos(x5)*sin(x5) + 2*x4*x6*mc*ml + 2*x4*x6*mc*mt + 2*x4*x6*ml*mt - Dt*x6*mc^2*sin(x5)^2 - 2*x4*x6*mc^2*cos(x5)^2 - 2*x4*x6*mc^2*sin(x5)^2 + bt*x2*mc*cos(x5) + bt*x2*ml*cos(x5) + g*mc*ml*sin(x5) + g*mc*mt*sin(x5) + g*ml*mt*sin(x5) - g*mc^2*cos(x5)^2*sin(x5) + Dt*x6*mc*ml + Dt*x6*mc*mt + Dt*x6*ml*mt - x6^2*x3*mc^2*cos(x5)*sin(x5) - 2*x4*x6*mc*ml*cos(x5)^2 + br*x4*mc*cos(x5)*sin(x5) + x6^2*x3*mc*ml*cos(x5)*sin(x5))/(x3*(mc*ml + mc*mt + ml*mt - mc^2*cos(x5)^2 - mc^2*sin(x5)^2 + mc^2 - mc*ml*cos(x5)^2));

== matlab function PSO_ZVD/non linear model/Model_Baocao1/Crane ==
  data: d1x input; l input; d1l input; the input; dx1 output; d1the input; Fx input; Fl input; dx2 output; dx3 output; dx4 output; dx5 output; dx6 output; bc input; mp input
function [dx1,dx2,dx3,dx4,dx5,dx6] = fcn(d1x,l,d1l,the,d1the,Fx,Fl,bc,mp)
 mt =5; mh =2; bt =0; br =0;  g =9.81;
 %bt =20; br =50;

dx1 = d1x;

%dx2 = (Fx*l*mh + Fx*l*mp - Fl*l*mp*sin(the) + bc*d1the*mh*cos(the) + bc*d1the*mp*cos(the) - d1the^2*l^2*mp^2*sin(the) + d1x^2*l^2*mp^2*sin(the) - bt*d1x*l*mh - bt*d1x*l*mp + d1x^2*l^2*mh*mp*sin(the) + br*d1l*l*mp*sin(the) + g*l*mh*mp*cos(the)*sin(the))/(l*(mh*mp + mh*mt + mp*mt - mp^2*cos(the)^2 - mp^2*sin(the)^2 + mp^2 - mh*mp*cos(the)^2));
dx2=(Fx*mh + Fx*mp - Fl*mp*sin(the) - d1the^2*l*mp^2*sin(the) + d1x^2*l*mp^2*sin(the) + d1x^2*l*mh*mp*sin(the) + g*mh*mp*cos(the)*sin(the))/(mh*mp + mh*mt + mp*mt - mp^2*cos(the)^2 - mp^2*sin(the)^2 + mp^2 - mh*mp*cos(the)^2); 

dx3 = d1l;

%dx4 = -(d1x^2*l^2*mp^2*sin(the)^2 - Fl*l*mt - d1the^2*l^2*mp^2 - Fl*l*mp + g*l*mp^2*cos(the)^3 + Fx*l*mp*sin(the) + Fl*l*mp*cos(the)^2 - d1the^2*l^2*mp*mt - g*l*mp^2*cos(the) + d1the^2*l^2*mp^2*cos(the)^2 + br*d1l*l*mp + br*d1l*l*mt + g*l*mp^2*cos(the)*sin(the)^2 - br*d1l*l*mp*cos(the)^2 + bc*d1the*mp*cos(the)*sin(the) - g*l*mp*mt*cos(the) - bt*d1x*l*mp*sin(the))/(l*(mh*mp + mh*mt + mp*mt - mp^2*cos(the)^2 - mp^2*sin(the)^2 + mp^2 - mh*mp*cos(the)^2));
dx4=(- l*d1the^2*mp^2*cos(the)^2 + l*d1the^2*mp^2 + l*mt*d1the^2*mp - l*d1x^2*mp^2*sin(the)^2 - g*mp^2*cos(the)^3 - g*mp^2*cos(the)*sin(the)^2 + g*mp^2*cos(the) - Fl*mp*cos(the)^2 + g*mt*mp*cos(the) - Fx*mp*sin(the) + Fl*mp + Fl*mt)/(mh*mp + mh*mt + mp*mt - mp^2*cos(the)^2 - mp^2*sin(the)^2 + mp^2 - mh*mp*cos(the)^2);

dx5 = d1the;

%dx6 = -(bc*d1the*mp^2 + bc*d1the*mh*mp + bc*d1the*mh*mt + bc*d1the*mp*mt - bc*d1the*mp^2*sin(the)^2 - g*l*mp^3*sin(the)^3 + 2*d1l*d1the*l*mp^3 + Fx*l*mp^2*cos(the) + g*l*mp^3*sin(the) - g*l*mp^3*cos(the)^2*sin(the) - bt*d1x*l*mp^2*cos(the) + g*l*mh*mp^2*sin(the) + g*l*mp^2*mt*sin(the) - d1the^2*l^2*mp^3*cos(the)*sin(the) + d1x^2*l^2*mp^3*cos(the)*sin(the) - 2*d1l*d1the*l*mp^3*cos(the)^2 - Fl*l*mp^2*cos(the)*sin(the) - 2*d1l*d1the*l*mp^3*sin(the)^2 + Fx*l*mh*mp*cos(the) + 2*d1l*d1the*l*mh*mp^2 + 2*d1l*d1the*l*mp^2*mt - 2*d1l*d1the*l*mh*mp^2*cos(the)^2 + br*d1l*l*mp^2*cos(the)*sin(the) - bt*d1x*l*mh*mp*cos(the) + g*l*mh*mp*mt*sin(the) + 2*d1l*d1the*l*mh*mp*mt + d1x^2*l^2*mh*mp^2*cos(the)*sin(the))/(l^2*mp*(mh*mp + mh*mt + mp*mt - mp^2*cos(the)^2 - mp^2*sin(the)^2 + mp^2 - mh*mp*cos(the)^2));
dx6=-(g*mp^2*sin(the) - g*mp^2*sin(the)^3 + Fx*mh*cos(the) + Fx*mp*cos(the) + 2*d1l*d1the*mp^2 + 2*d1l*d1the*mh*mp + 2*d1l*d1the*mh*mt + 2*d1l*d1the*mp*mt - 2*d1l*d1the*mp^2*cos(the)^2 - 2*d1l*d1the*mp^2*sin(the)^2 + g*mh*mp*sin(the) + g*mh*mt*sin(the) + g*mp*mt*sin(the) - g*mp^2*cos(the)^2*sin(the) - Fl*mp*cos(the)*sin(the) - d1the^2*l*mp^2*cos(the)*sin(the) + d1x^2*l*mp^2*cos(the)*sin(the) - 2*d1l*d1the*mh*mp*cos(the)^2 + d1x^2*l*mh*mp*cos(the)*sin(the))/(l*(mh*mp + mh*mt + mp*mt - mp^2*cos(the)^2 - mp^2*sin(the)^2 + mp^2 - mh*mp*cos(the)^2));

== matlab function PSO_ZVD/non linear model/enhanced/Crane ==
  data: dx1 output; d1x input; the1 input; d1the1 input; the2 input; d1the2 input; Fx input; dx2 output; dx3 output; dx4 output; dx5 output; dx6 output; m2 input; m input; m1 input
function [dx1,dx2,dx3,dx4,dx5,dx6] = fcn(d1x,the1,d1the1,the2,d1the2,Fx,m2,m,m1)
g =9.81; l2=0.5; l1=0.1;
 %bx=20; bl=50;

 dx1=d1x;

 dx2 = -(Fx*m1 + Fx*m2 - Fx*m2*cos(the1 - the2)^2 + d1the1^2*l1*m1^2*sin(the1) + d1the1^2*l1*m2^2*sin(the1) + d1the2^2*l2*m2^2*sin(the2) + g*m1^2*cos(the1)*sin(the1) + g*m2^2*cos(the1)*sin(the1) + g*m2^2*cos(the2)*sin(the2) - d1the1^2*l1*m2^2*sin(the1 - the2)*cos(the2) + d1the2^2*l2*m2^2*sin(the1 - the2)*cos(the1) + 2*d1the1^2*l1*m1*m2*sin(the1) + d1the2^2*l2*m1*m2*sin(the2) - g*m2^2*cos(the1 - the2)*cos(the1)*sin(the2) - g*m2^2*cos(the1 - the2)*cos(the2)*sin(the1) + 2*g*m1*m2*cos(the1)*sin(the1) + g*m1*m2*cos(the2)*sin(the2) - d1the1^2*l1*m2^2*cos(the1 - the2)^2*sin(the1) - d1the2^2*l2*m2^2*cos(the1 - the2)^2*sin(the2) + d1the1^2*l1*m2^2*cos(the1 - the2)*sin(the1 - the2)*cos(the1) - d1the2^2*l2*m2^2*cos(the1 - the2)*sin(the1 - the2)*cos(the2) - d1the1^2*l1*m1*m2*sin(the1 - the2)*cos(the2) + d1the2^2*l2*m1*m2*sin(the1 - the2)*cos(the1) - g*m1*m2*cos(the1 - the2)*cos(the1)*sin(the2) - g*m1*m2*cos(the1 - the2)*cos(the2)*sin(the1) - d1the1^2*l1*m1*m2*cos(the1 - the2)^2*sin(the1) + d1the1^2*l1*m1*m2*cos(the1 - the2)*sin(the1 - the2)*cos(the1))/(m1^2*cos(the1)^2 - m*m2 - 2*m1*m2 - m*m1 + m2^2*cos(the1)^2 + m2^2*cos(the2)^2 + m2^2*cos(the1 - the2)^2 - m1^2 - m2^2 + 2*m1*m2*cos(the1)^2 + m1*m2*cos(the2)^2 + m*m2*cos(the1 - the2)^2 + m1*m2*cos(the1 - the2)^2 - 2*m2^2*cos(the1 - the2)*cos(the1)*cos(the2) - 2*m1*m2*cos(the1 - the2)*cos(the1)*cos(the2));

 dx3=d1the1;

 dx4 = (g*m1^2*sin(the1) + g*m2^2*sin(the1) + Fx*m1*cos(the1) + Fx*m2*cos(the1) + d1the2^2*l2*m2^2*sin(the1 - the2) - g*m2^2*cos(the1 - the2)*sin(the2) + g*m*m1*sin(the1) + g*m*m2*sin(the1) + 2*g*m1*m2*sin(the1) - g*m2^2*cos(the2)^2*sin(the1) - Fx*m2*cos(the1 - the2)*cos(the2) + d1the1^2*l1*m1^2*cos(the1)*sin(the1) + d1the1^2*l1*m2^2*cos(the1)*sin(the1) + d1the2^2*l2*m2^2*cos(the1)*sin(the2) + g*m2^2*cos(the1)*cos(the2)*sin(the2) + d1the1^2*l1*m2^2*cos(the1 - the2)*sin(the1 - the2) + d1the2^2*l2*m*m2*sin(the1 - the2) + d1the2^2*l2*m1*m2*sin(the1 - the2) - g*m*m2*cos(the1 - the2)*sin(the2) - g*m1*m2*cos(the1 - the2)*sin(the2) - d1the2^2*l2*m2^2*sin(the1 - the2)*cos(the2)^2 - g*m1*m2*cos(the2)^2*sin(the1) - d1the1^2*l1*m2^2*cos(the1 - the2)*cos(the2)*sin(the1) - d1the1^2*l1*m2^2*sin(the1 - the2)*cos(the1)*cos(the2) - d1the2^2*l2*m2^2*cos(the1 - the2)*cos(the2)*sin(the2) + 2*d1the1^2*l1*m1*m2*cos(the1)*sin(the1) + d1the2^2*l2*m1*m2*cos(the1)*sin(the2) + g*m1*m2*cos(the1)*cos(the2)*sin(the2) + d1the1^2*l1*m*m2*cos(the1 - the2)*sin(the1 - the2) + d1the1^2*l1*m1*m2*cos(the1 - the2)*sin(the1 - the2) - d1the1^2*l1*m1*m2*cos(the1 - the2)*cos(the2)*sin(the1) - d1the1^2*l1*m1*m2*sin(the1 - the2)*cos(the1)*cos(the2))/(l1*(m1^2*cos(the1)^2 - m*m2 - 2*m1*m2 - m*m1 + m2^2*cos(the1)^2 + m2^2*cos(the2)^2 + m2^2*cos(the1 - the2)^2 - m1^2 - m2^2 + 2*m1*m2*cos(the1)^2 + m1*m2*cos(the2)^2 + m*m2*cos(the1 - the2)^2 + m1*m2*cos(the1 - the2)^2 - 2*m2^2*cos(the1 - the2)*cos(the1)*cos(the2) - 2*m1*m2*cos(the1 - the2)*cos(the1)*cos(the2)));

 dx5=d1the2;

 dx6 = -(d1the1^2*l1*m1^2*sin(the1 - the2) - g*m2^2*sin(the2) - Fx*m1*cos(the2) - Fx*m2*cos(the2) - g*m1^2*sin(the2) + d1the1^2*l1*m2^2*sin(the1 - the2) + g*m1^2*cos(the1 - the2)*sin(the1) + g*m2^2*cos(the1 - the2)*sin(the1) - g*m*m1*sin(the2) - g*m*m2*sin(the2) - 2*g*m1*m2*sin(the2) + g*m1^2*cos(the1)^2*sin(the2) + g*m2^2*cos(the1)^2*sin(the2) + Fx*m1*cos(the1 - the2)*cos(the1) + Fx*m2*cos(the1 - the2)*cos(the1) - d1the1^2*l1*m1^2*cos(the2)*sin(the1) - d1the1^2*l1*m2^2*cos(the2)*sin(the1) - d1the2^2*l2*m2^2*cos(the2)*sin(the2) - g*m1^2*cos(the1)*cos(the2)*sin(the1) - g*m2^2*cos(the1)*cos(the2)*sin(the1) + d1the2^2*l2*m2^2*cos(the1 - the2)*sin(the1 - the2) + d1the1^2*l1*m*m1*sin(the1 - the2) + d1the1^2*l1*m*m2*sin(the1 - the2) + 2*d1the1^2*l1*m1*m2*sin(the1 - the2) + g*m*m1*cos(the1 - the2)*sin(the1) + g*m*m2*cos(the1 - the2)*sin(the1) + 2*g*m1*m2*cos(the1 - the2)*sin(the1) - d1the1^2*l1*m1^2*sin(the1 - the2)*cos(the1)^2 - d1the1^2*l1*m2^2*sin(the1 - the2)*cos(the1)^2 + 2*g*m1*m2*cos(the1)^2*sin(the2) + d1the1^2*l1*m1^2*cos(the1 - the2)*cos(the1)*sin(the1) + d1the1^2*l1*m2^2*cos(the1 - the2)*cos(the1)*sin(the1) + d1the2^2*l2*m2^2*cos(the1 - the2)*cos(the1)*sin(the2) - d1the2^2*l2*m2^2*sin(the1 - the2)*cos(the1)*cos(the2) - 2*d1the1^2*l1*m1*m2*cos(the2)*sin(the1) - d1the2^2*l2*m1*m2*cos(the2)*sin(the2) - 2*g*m1*m2*cos(the1)*cos(the2)*sin(the1) + d1the2^2*l2*m*m2*cos(the1 - the2)*sin(the1 - the2) + d1the2^2*l2*m1*m2*cos(the1 - the2)*sin(the1 - the2) - 2*d1the1^2*l1*m1*m2*sin(the1 - the2)*cos(the1)^2 + 2*d1the1^2*l1*m1*m2*cos(the1 - the2)*cos(the1)*sin(the1) + d1the2^2*l2*m1*m2*cos(the1 - the2)*cos(the1)*sin(the2) - d1the2^2*l2*m1*m2*sin(the1 - the2)*cos(the1)*cos(the2))/(l2*(m1^2*cos(the1)^2 - m*m2 - 2*m1*m2 - m*m1 + m2^2*cos(the1)^2 + m2^2*cos(the2)^2 + m2^2*cos(the1 - the2)^2 - m1^2 - m2^2 + 2*m1*m2*cos(the1)^2 + m1*m2*cos(the2)^2 + m*m2*cos(the1 - the2)^2 + m1*m2*cos(the1 - the2)^2 - 2*m2^2*cos(the1 - the2)*cos(the1)*cos(the2) - 2*m1*m2*cos(the1 - the2)*cos(the1)*cos(the2)));
